simulink model "sm_parts_circ_tubes"  (R2026a)
settings: Solver=VariableStepAuto  EnableMultiTasking=on
libraries: Multibody_Parts_Lib x3, sm_lib x2, nesl_utility x1
Description:
  | Copyright 2017-2026 The MathWorks, Inc.
settings Model: Creator=smiller  LastModifiedBy=smiller
settings DebuggingCC: PregeneratedLibrarySubsystemCodeDiagnostic=none
settings SimscapeCC: SimscapeNormalizeSystem=off  SimscapeNominalValues="[{\"value\":\"1\",\"unit\":\"A\"},{\"value\":\"1\",\"unit\":\"bar\"},{\"value\":\"1\",\"unit\":\"cm^2\"},{\"value\":\"1\",\"unit\":\"cm^3/s\"},{\"value\":\"1\",\"unit\":\"kJ/kg\"},{\"value\":\"1\",\"unit\":\"kW\"},{\"value\":\"1\",\"unit\":\"l\"},{\"value\":\"1\",\"unit\":\"N\"},{\"value\":\"1\",\"unit\":\"N*m\"},{\"value\":\"1\",\"unit\":\"V\"}]"
settings ConfigurationSet: Description=SimMechanics 2G
settings ExplorerConfigSet: InternalSimMechanicsExplorerSettings="<ExplorerConfiguration><canonicalview>default</canonicalview><AnimationSetting><BasePlaybackSpeed>1.0</BasePlaybackSpeed><PlaybackSpeedFactor>1.0</PlaybackSpeedFactor></AnimationSetting><TilePanel><TileInfo><Tiles Columns=\"1\" Count=\"1\" Rows=\"1\"><Column Left=\"2\" Weight=\"1\"/><Column Left=\"429\"/><Row Top=\"2\" Weight=\"1\"/><Row Top=\"206\"/><Tile Height=\"1\" Width=\"1\" X=\"0\" Y=\"0\"/></Tiles></TileInfo><SceneInfo><SceneViewer><BGColor><R>1</R><G>1</G><B>1</B></BGColor><Camera><DoPerspective>off</DoPerspective><Position><X>0.56604864133702248</X><Y>0.20706989406685108</Y><Z>-0.47573574864511947</Z></Position><Center><X>-0.39392450478888347</X><Y>0.11157273285489984</Y><Z>-0.21242632815738077</Z></Center><Up><X>-0.088140973552186155</X><Y>0.99531902580127296</Y><Z>0.039638436640211092</Z></Up><ViewLimDist>1</ViewLimDist><YLim>0.24687643915414811</YLim><XLim>0.52920180290478924</XLim></Camera></SceneViewer></SceneInfo></TilePanel><MechEditorPanel><Cameras/><GfxPanelCameraMap/><VideoCreator><PlaybackSpeedRatio>1.0</PlaybackSpeedRatio><FrameRate>30</FrameRate><VideoFormat>Motion JPEG AVI</VideoFormat><FrameSize>auto</FrameSize></VideoCreator></MechEditorPanel></ExplorerConfiguration>"

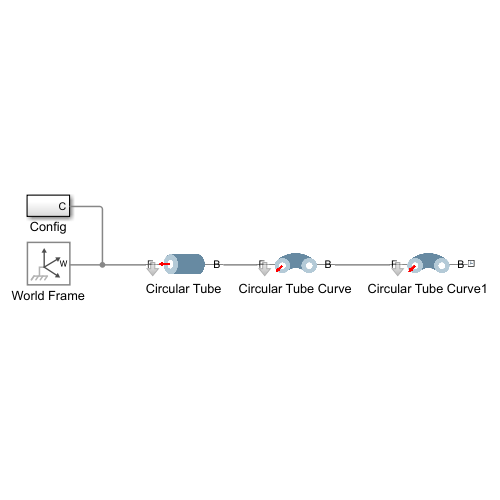
[thumbnail: Simulink's stored preview of the top-level diagram]
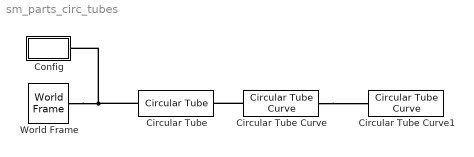
== system sm_parts_circ_tubes ==
  Circular Tube : Multibody_Parts_Lib/Extrusions/Circular Tube  circ_radout=10e-2  circ_radin=5e-2  deg_1=45  deg_2=315  circ_len=0.3  circ_rho=7000  circ_color=[0 0.4 0.6]  circ_opc=1
      settings: SourceProductName=Simscape Multibody Parts Library
  Circular Tube Curve : Multibody_Parts_Lib/Extrusions/Circular Tube Curve  circ_radout=10e-2  circ_radin=5e-2  deg_1=45  deg_2=315  arc_rad=0.25  arc_angle=115  popup_arcdir=Y  circ_rho=7000  circ_color=[0.8 0.8 0.8]  circ_opc=1
      settings: SourceProductName=Simscape Multibody Parts Library
  Circular Tube Curve1 : Multibody_Parts_Lib/Extrusions/Circular Tube Curve  circ_radout=10e-2  circ_radin=5e-2  deg_1=45  deg_2=315  arc_rad=12e-2  arc_angle=180  popup_arcdir=Z  circ_rho=7000  circ_color=[0 0.4 0.6]  circ_opc=1
      settings: SourceProductName=Simscape Multibody Parts Library
  Config : Subsystem
  World Frame : sm_lib/Frames and Transforms/World Frame
  connections:
  World Frame/RConn1 -- Config/LConn1 -- Circular Tube/RConn1
  Circular Tube Curve/RConn1 -- Circular Tube/LConn1
  Circular Tube Curve/LConn1 -- Circular Tube Curve1/RConn1

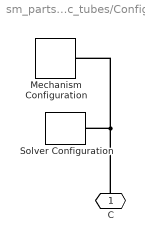
== system sm_parts_circ_tubes/Config ==
  Mechanism Configuration : sm_lib/Utilities/Mechanism Configuration  UniformGravity=Constant  GravityVector=[0 0 -9.80665]  GravityVectorUnits=m/s^2  LinearizationDelta=0.001  JointModeTransitionNonlinearIterations=2
  Solver Configuration : nesl_utility/Solver Configuration  PhysicalDomain=network_engine_domain  SubClassName=solver  LeftPortType=input  RightPortType=generic  Tones=[]  Harmonics=[]  SimulateNoise=off  Profile=off  UseLocalSampling=off  EnableSwitchedLinearOptims=on  FrequencyDomain=off  UseCCode=off  RelTol=0.001  AbsTol=1e-06  MinStep=1e-09  ToWorkspace=off  RevertToSquareIcSolve=off  NumHomotopyIterations=100  PhasorMode=off  PhasorModeNumHarmonics=1  ConsistencySolver=NEWTON_FTOL  CanonicalOrdering=UNORDERED  OptimizeIntermediates=UNOPTIMIZED  IndexReductionMethod=DerivativeReplacement  DoDC=off  ResidualTolerance=1e-09  ConsistencyTolSource=GLOBAL  ConsistencyAbsTol=0.001  ConsistencyRelTol=0.001  ConsistencyTolFactor=0.001  UseLocalSolver=off  LocalSolverChoice=NE_BACKWARD_EULER_ADVANCER  ResolveIndetEquations=on  FunctionEvalNumThread=1  LocalSolverSampleTime=0.001  DoFixedCost=off  MaxNonlinIter=3  MaxModeIter=2  ComputeImpulses=off  ImpulseIterations=2  LinearAlgebra=Sparse  LinearAlgebraNumThread=0  EquationFormulation=NE_TIME_EF  DelaysMemoryBudget=1024  AutomaticFiltering=on  FilteringTimeConstant=0.001  PartitionStorageMethod=AS_NEEDED  PartitionMemoryBudget=1024  PartitionMethod=FAST  MultibodyUseLocalSolver=off  MultibodyLocalSolverChoice=ODE1  MultibodyLocalSolverSampleTime=0.001
  C : PMIOPort  Side=Left
  connections:
  Mechanism Configuration/RConn1 -- C/RConn1 -- Solver Configuration/RConn1
